simulink model "ej0314_SimuControladores"  (R2019b)
settings: Solver=VariableStepAuto  StartTime=0.0  StopTime=10.0  RelTol=1e-3
values from neighbouring files (symbols this model uses):
  den = conv(conv([1 0],[1 6]),[1 18])    [ej0314_Controladores.m]    (also in ej0427_servoretrovelocidad.m = [1 2 0]; ej0509_unceroS3erorden.m = den{1}; ej0518_avion.m = [den 0])
  K1 = 0.45*Kcr    (= 1.08)    [ej0314_Controladores.m]
  K2 = 0.6*Kcr    (= 1.44)    [ej0314_Controladores.m]
  Kcr = 2.4    [ej0314_Controladores.m]
  num = 1080    [ej0314_Controladores.m]    (also in ej0427_servoretrovelocidad.m = 1; ej0509_unceroS3erorden.m = num{1}; ej0518_avion.m = double(num))
  Ti1 = Tcr/1.2    (= 0.503460361152)    [ej0314_Controladores.m]
  Ti2 = 0.5*Tcr    (= 0.302076216691)    [ej0314_Controladores.m]
settings Model: Creator=cjuar  LastModifiedBy=cjuar

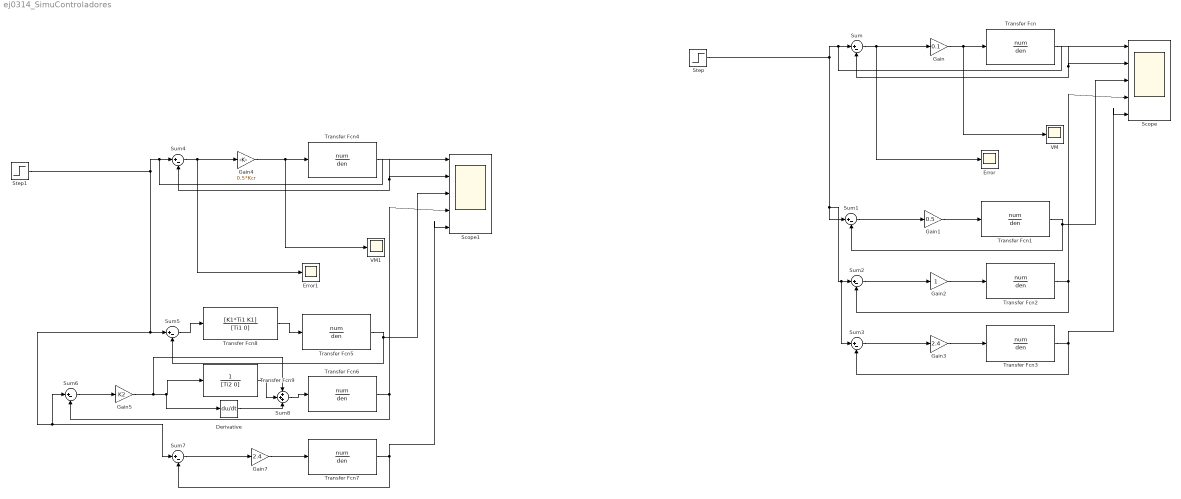
== system ej0314_SimuControladores ==
  Derivative : Derivative  CoefficientInTFapproximation=Td2
  Error : Scope
  Error1 : Scope
  Gain : Gain  Gain=0.1
  Gain1 : Gain  Gain=0.5
  Gain2 : Gain
  Gain3 : Gain  Gain=2.4
  Gain4 : Gain  Gain=0.5*Kcr
  Gain5 : Gain  Gain=K2
  Gain7 : Gain  Gain=2.4
  Scope : Scope  NumInputPorts=5
  Scope1 : Scope  NumInputPorts=5
  Step : Step  SampleTime=0
  Step1 : Step  SampleTime=0
  Sum{,1..7} (8 alike) : Sum  Inputs=|+-
  Sum8 : Sum  Inputs=+++
  Transfer Fcn{,1..7} (8 alike) : TransferFcn  Numerator=num  Denominator=den
  Transfer Fcn8 : TransferFcn  Numerator=[K1*Ti1 K1]  Denominator=[Ti1 0]
  Transfer Fcn9 : TransferFcn  Denominator=[Ti2 0]
  VM : Scope
  VM1 : Scope
  wires:
  Gain/1 -> VM/1, Transfer Fcn/1
  Transfer Fcn/1 -> Scope/2, Sum/2
  Sum/1 -> Error/1, Gain/1
  Transfer Fcn1/1 -> Scope/3, Sum1/2
  Sum1/1 -> Gain1/1
  Gain1/1 -> Transfer Fcn1/1
  Sum2/1 -> Gain2/1
  Gain2/1 -> Transfer Fcn2/1
  Transfer Fcn2/1 -> Sum2/2, Scope/4
  Sum3/1 -> Gain3/1
  Step/1 -> Scope/1, Sum/1, Sum3/1, Sum2/1, Sum1/1
  Gain3/1 -> Transfer Fcn3/1
  Transfer Fcn3/1 -> Sum3/2, Scope/5
  Step1/1 -> Scope1/1, Sum4/1, Sum7/1, Sum6/1, Sum5/1
  Transfer Fcn4/1 -> Scope1/2, Sum4/2
  Sum4/1 -> Error1/1, Gain4/1
  Gain4/1 -> VM1/1, Transfer Fcn4/1
  Transfer Fcn7/1 -> Sum7/2, Scope1/5
  Sum7/1 -> Gain7/1
  Sum5/1 -> Transfer Fcn8/1
  Gain7/1 -> Transfer Fcn7/1
  Transfer Fcn8/1 -> Transfer Fcn5/1
  Transfer Fcn6/1 -> Sum6/2, Scope1/4
  Transfer Fcn5/1 -> Scope1/3, Sum5/2
  Sum6/1 -> Gain5/1
  Gain5/1 -> Sum8/1, Derivative/1, Transfer Fcn9/1
  Derivative/1 -> Sum8/3
  Transfer Fcn9/1 -> Sum8/2
  Sum8/1 -> Transfer Fcn6/1
